simulink model "P2001_230205_InstantaneousCostEM1"  (R2022b)
settings: Solver=VariableStepAuto  StartTime=0.0  StopTime=30  RelTol=1e-7
settings Model: PacingRate=0.110000  Creator=turib  LastModifiedBy=turib
settings HardwareCC: ProdHWDeviceType=AMD->x86-64 (Windows64)

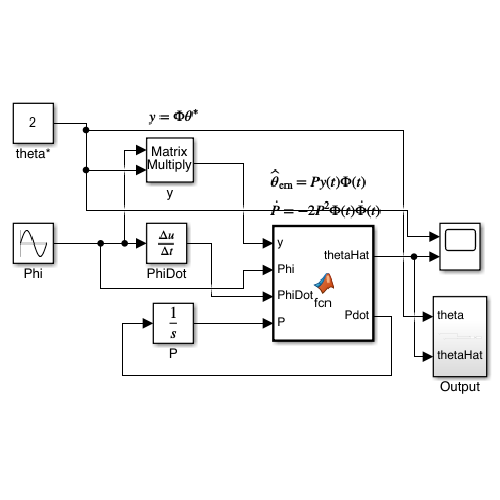
[thumbnail: Simulink's stored preview of the top-level diagram]
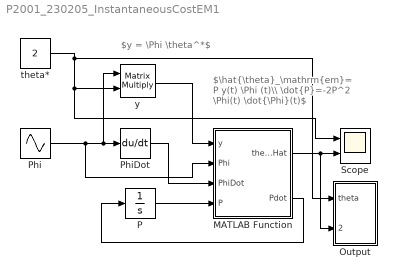
== system P2001_230205_InstantaneousCostEM1 ==
  note: $y = \Phi \theta^*$
  note: $\hat{\theta}_\mathrm{em}= P y(t) \Phi (t)\\ \dot{P}=-2P^2 \Phi(t) \dot{\Phi}(t)$
  MATLAB Function : MATLAB Function  TreatAsAtomicUnit=on
  Output : Subsystem
  P : Integrator  InitialCondition=1
  Phi : Sin  SampleTime=0
  PhiDot : Derivative
  Scope : Scope  NumInputPorts=2
  theta* : Constant  Value=2
  y : Product  Multiplication=Matrix(*)  OutDataTypeStr=double
  wires:
  theta*/1 -> y/2, Scope/1, Output/1(theta)
  Phi/1 -> PhiDot/1, y/1, MATLAB Function/2(Phi)
  PhiDot/1 -> MATLAB Function/3(PhiDot)
  y/1 -> MATLAB Function/1(y)
  P/1 -> MATLAB Function/4(P)
  MATLAB Function/1(thetaHat) -> Output/2(thetaHat), Scope/2
  MATLAB Function/2(Pdot) -> P/1

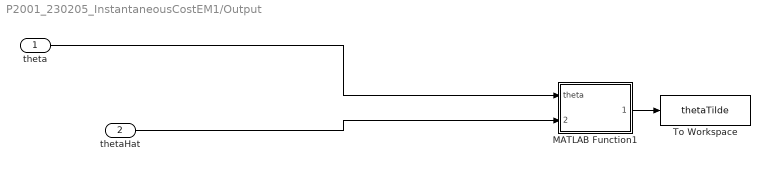
== system P2001_230205_InstantaneousCostEM1/Output ==
  theta : Inport
  thetaHat : Inport  Port=2
  MATLAB Function1 : MATLAB Function  TreatAsAtomicUnit=on
  To Workspace : ToWorkspace  VariableName=thetaTilde  SampleTime=-1
  wires:
  MATLAB Function1/1(thetaTilde) -> To Workspace/1
  thetaHat/1 -> MATLAB Function1/2(thetaHat)
  theta/1 -> MATLAB Function1/1(theta)

== matlab function P2001_230205_InstantaneousCostEM1/Output/MATLAB Function1 ==
  data: theta input; thetaTilde output; thetaHat input
function thetaTilde = error(theta, thetaHat)

thetaTilde = thetaHat - theta;

end

== matlab function P2001_230205_InstantaneousCostEM1/MATLAB Function ==
  data: thetaHat output; y input; Phi input; PhiDot input; Pdot output; P input
function [thetaHat, Pdot] = fcn(y, Phi, PhiDot, P)
thetaHat = P * y * Phi;
Pdot = - 2 * (P ^ 2) * Phi * PhiDot;
end
